simulink model "Transfer"  (R2025a)
settings: Solver=VariableStepAuto  StartTime=0.0  StopTime=5  RelTol=1e-3
settings Model: Creator=cruisemac  LastModifiedBy=cruisemac

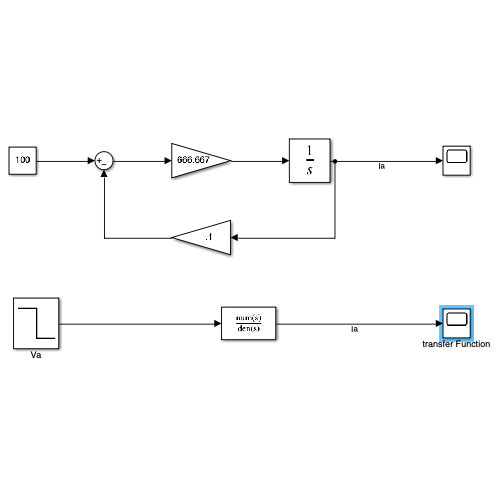
[thumbnail: Simulink's stored preview of the top-level diagram]
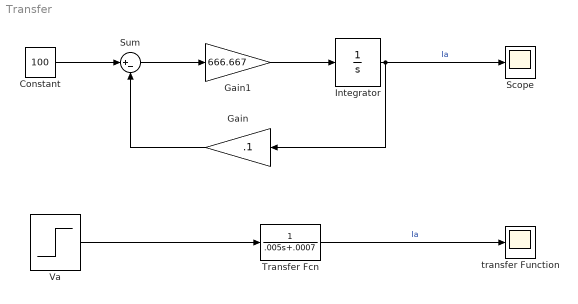
== system Transfer ==
  Constant : Constant  Value=100
  Gain : Gain  Gain=.1
  Gain1 : Gain  Gain=666.667
  Integrator : Integrator
  Scope : Scope
      settings: ActiveDisplayYMinimum=625.8905578416036  ActiveDisplayYMaximum=633.94153295739955
  Sum : Sum  Inputs=|+-
  Transfer Fcn : TransferFcn  Denominator=[.005 .0007]
  Va : Step  Time=2  Before=1  After=0  SampleTime=0
  transfer Function : Scope
      settings: ActiveDisplayYMinimum=-3.8820282376771331  ActiveDisplayYMaximum=439.4460516758885
  wires:
  Sum/1 -> Gain1/1
  Gain1/1 -> Integrator/1
  Integrator/1 -> Scope/1, Gain/1  "Ia"
  Gain/1 -> Sum/2
  Transfer Fcn/1 -> transfer Function/1  "Ia"
  Constant/1 -> Sum/1
  Va/1 -> Transfer Fcn/1
